simulink library "ddm"  (R2021b)
settings: Solver=VariableStepAuto  StartTime=0.0  StopTime=10.0  RelTol=1e-3
undefined symbols (not defined in the file or in its folder): ENUM_ADASACCSTA_ERROR, ENUM_ADASACCSTA_OFF, ENUM_ADASACCSTA_STANDBY, ENUM_ADASISASTA_OFF, ENUM_ALLOWMOV_ALLOWREADY, ENUM_APS, ENUM_BRKSTA_ERROR, ENUM_BRKSTA_OFF, ENUM_BRKSTA_ON, ENUM_BRKSW_INVALID, ENUM_BRKSW_OFF, ENUM_BRKSW_ON, ENUM_CHGPREACTERRSTA_OBCPRE, ENUM_DCDCFAULTSTA_ANYFAULTLV1, ENUM_DCDCFAULTSTA_ANYFAULTLV2, ENUM_DRIVETRAIN_AWD, ENUM_DRIVETRAIN_FWD, ENUM_DRIVETRAIN_RWD, ENUM_DRSEATSTA_INVALID, ENUM_EDUDRTSTA_NORMAL, ENUM_EPBSTA_APPLIED, ENUM_EPBSTA_RELEASED, ENUM_HVBATTREADYPRE_READY, ENUM_MCUWARN_LV0, ENUM_MCUWARN_LV1, ENUM_MCUWARN_LV2, ENUM_MCUWARN_LV3, ENUM_MCUWARN_NOERROR, ENUM_OBCFAULTSTA_ANYFAULT, ENUM_PAS_R2F2, ENUM_PDFAULT_BATTPDFAIL, ENUM_PDFAULT_DCDCDISABLE, ENUM_PDFAULT_MCUDISABLE, ENUM_PDFAULT_MCUDISCHRG, ENUM_POWERSTA_OFF, ENUM_POWERSTA_ON, ENUM_POWERSTA_READY, ENUM_POWERSTA_STANDBY, ENUM_PRESSINDI_LOW, ENUM_PUFAULT_BATTUPFAIL, ENUM_PUFAULT_DCDCENABLEFAIL, ENUM_PUFAULT_PRECHRGCHKFAIL, ENUM_PUFAULT_SAFETYCHKFAIL, ENUM_PUSTATE_COMPLETED, ENUM_PWRSTASW_OFF, ENUM_PWRSTASW_OFFA, ENUM_PWRSTASW_OFFCHVCHRG, ENUM_PWRSTASW_OFFCLVCHRG, ENUM_PWRSTASW_ON, ENUM_PWRSTASW_ONHVCHRG, ENUM_PWRSTASW_READY, ENUM_PWRSTASW_STANDBY, ENUM_RANGESTA_12IN, ENUM_SHIFTCOMMAND_D, ENUM_SHIFTCOMMAND_N, ENUM_SHIFTCOMMAND_P, ENUM_SHIFTCOMMAND_R, ENUM_VEHMALFUNLV_2ND, ENUM_VEHMALFUNLV_3RD, ENUM_VEHMALFUNLV_4TH ... (+835)
libraries: hcu_lib x750, $bdroot x12, simulink x5
(part 18 of 28)

== system ddm/DDM/DDM/PMM/Fault level/Fault level 1 subsystem error ==
  note: Diagnostics and Fault Handling
  note: Release Condition After Failure Decision
  note: Test Detection Criteria
  note: Test Pass Criteria
  note: Fail Safe Operation After Failure Decision
  note: Release Condition During Failure Detection
  note: Fail Safe Operation During Failure Detection
  task_time_s : Inport
  VPMM_PowerSta_enum : Inport  Port=2
  VPMM_PwrStaSW_enum : Inport  Port=3
  VDDM_C3BMS6LCCFS_flg : Inport  Port=4
  VDDM_C3CCU2LCCFS_flg : Inport  Port=5
  VDDM_MCUF1NoComCFS_flg : Inport  Port=6
  VDDM_MCUR1NoComCFS_flg : Inport  Port=7
  VINP_BMSWarn1_flg : Inport  Port=8
  VINP_BMSWarn2_flg : Inport  Port=9
  VINP_BMSWarn3_flg : Inport  Port=10
  VINP_DCDCFaultSta_enum : Inport  Port=11
  VINP_MCUWarnF_enum : Inport  Port=12
  VINP_MCUWarnR_enum : Inport  Port=13
  VINP_OBCFaultSta_enum : Inport  Port=14
  VPMM_DrivetrainSelect_enum : Inport  Port=15
  DTC_clear_request : Inport  Port=16
  No_CAN3_BUS_OFF : Inport  Port=17
  Constant : Constant  Value=KDDM_Lv1ErrDetTO_s
  Constant1 : Constant  Value=KDDM_Lv1ErrPassTO_s
  Constant{5,10,42,47} (4 alike) : Constant  Value=ENUM_MCUWARN_LV0
  Constant{6,11,43,49} (4 alike) : Constant  Value=ENUM_DRIVETRAIN_AWD
  Constant12 : Constant  Value=KDDM_Lv1ErrDTC_cnt
  Constant13 : Constant  Value=KDDM_Lv1ErrDetSW_flg
  Constant14 : Constant  Value=KDDM_Lv1ErrPassSW_flg
  Constant{15,21,25,27} (4 alike) : Constant  Value=FALSE
  Constant18 : Constant  Value=KDDM_Lv1ErrPassTO_s
  Constant2 : Constant  Value=KDDM_Lv1ErrCFSSW_flg
  Constant24 : Constant  Value=TRUE
  Constant26 : Constant  Value=ENUM_PWRSTASW_OFF
  Constant3 : Constant  Value=TRUE
  Constant36 : Constant  Value=ENUM_DCDCFAULTSTA_ANYFAULTLV1
  Constant37 : Constant  Value=ENUM_OBCFAULTSTA_ANYFAULT
  Constant38 : Constant  Value=ENUM_PWRSTASW_OFF
  Constant39 : Constant  Value=TRUE
  Constant4 : Constant  Value=ENUM_POWERSTA_OFF
  Constant40 : Constant  Value=KDDM_Lv1ErrDTC_cnt
  Constant44 : Constant  Value=ENUM_DRIVETRAIN_FWD
  Constant45 : Constant  Value=ENUM_DRIVETRAIN_RWD
  Constant50 : Constant  Value=ENUM_DCDCFAULTSTA_ANYFAULTLV1
  Constant51 : Constant  Value=ENUM_OBCFAULTSTA_ANYFAULT
  Constant7 : Constant  Value=ENUM_DRIVETRAIN_FWD
  Constant8 : Constant  Value=ENUM_DRIVETRAIN_RWD
  Constant9 : Constant  Value=KDDM_Lv1ErrDFSSW_flg
  DTC_Couter : hcu_lib/Basic_Blocks/DTC_Couter
  DTC_Info : hcu_lib/Basic_Blocks/DTC_Info
  Data Type Conversion1 : DataTypeConversion  OutDataTypeStr=uint8
  Equal : RelationalOperator  Operator=~=  OutDataTypeStr=boolean  RndMeth=Simplest
  Equal{1,4..9,14..21,25..26} (17 alike) : RelationalOperator  Operator===  OutDataTypeStr=boolean  RndMeth=Simplest
  Equal2 : RelationalOperator  Operator=~=  OutDataTypeStr=boolean  RndMeth=Simplest
  Equal3 : RelationalOperator  OutDataTypeStr=boolean  RndMeth=Simplest
  Goto24 : Goto  Commented=on  GotoTag=VDDM_EDriveSysErrVCUErr_flg
  Logical Operator{1,4..7,9..10,21,27..28} (10 alike) : Logic  Operator=NOT  AllPortsSameDT=off  OutDataTypeStr=boolean
  Logical Operator11 : Logic  Operator=OR  Inputs=7  AllPortsSameDT=off  OutDataTypeStr=boolean
  Logical Operator{12..13,15..16,18,22,24} (7 alike) : Logic  AllPortsSameDT=off  OutDataTypeStr=boolean
  Logical Operator{8,14,17,23,25,29..30} (7 alike) : Logic  Operator=OR  AllPortsSameDT=off  OutDataTypeStr=boolean
  Logical Operator19 : Logic  Inputs=3  AllPortsSameDT=off  OutDataTypeStr=boolean
  Logical Operator2 : Logic  Inputs=6  AllPortsSameDT=off  OutDataTypeStr=boolean
  Logical Operator20 : Logic  Operator=OR  Inputs=7  AllPortsSameDT=off  OutDataTypeStr=boolean
  Logical Operator26 : Logic  Inputs=6  AllPortsSameDT=off  OutDataTypeStr=boolean
  Logical Operator3 : Logic  Operator=OR  Inputs=3  AllPortsSameDT=off  OutDataTypeStr=boolean
  Relay : Relay  OnSwitchValue=ONE_INT  OffSwitchValue=ZERO_INT
  SR_Latch1 : Subsystem  mask(SR_Latch){}
      mask help: SR latch function.
  SR_Latch3 : hcu_lib/Basic_Blocks/SR_Latch
  SR_Latch4 : hcu_lib/Basic_Blocks/SR_Latch
  Switch{,2,4..6} (5 alike) : Switch  Criteria=u2 ~= 0
  Test Detection Criteria : hcu_lib/Basic_Blocks/Test Detection Criteria
  Timer1 : hcu_lib/Basic_Blocks/Timer
  VDDM_Lv1ErrDTC_raw32 : Outport
  wires:
  Logical Operator12/1 -> [VDDM_Lv1ErrDFS_flg]  "VDDM_Lv1ErrDFS_flg"
  Constant12/1 -> DTC_Couter/3
  Constant14/1 -> Logical Operator15/2
  Constant2/1 -> Logical Operator18/2
  DTC_Couter/1 -> SR_Latch4/1
  [VDDM_Lv1ErrDet_flg] -> Logical Operator19/1
  [DTC_clear_request] -> Logical Operator3/3
  Logical Operator18/1 -> [VDDM_Lv1ErrCFS_flg]  "VDDM_Lv1ErrCFS_flg"
  [DTC_clear_request] -> Logical Operator21/1
  [VDDM_Lv1ErrCFSRls_flg] -> Logical Operator29/1
  SR_Latch4/1 -> Logical Operator18/1
  [VDDM_Lv1ErrPass_flg] -> Logical Operator3/1
  DTC_Couter/2 -> Data Type Conversion1/1
  Logical Operator21/1 -> Logical Operator19/3
  Relay/1 -> SR_Latch3/1
  Data Type Conversion1/1 -> [VDDM_Lv1ErrDTC_cnt]  "VDDM_Lv1ErrDTC_cnt"
  Logical Operator15/1 -> DTC_Couter/2
  [VDDM_Lv1ErrCFSRls_flg] -> Logical Operator3/2
  Logical Operator30/1 -> SR_Latch3/2
  [VDDM_Lv1ErrCFS_flg] -> Logical Operator30/1
  Logical Operator29/1 -> SR_Latch4/2
  Logical Operator3/1 -> Logical Operator15/1
  [DTC_clear_request] -> Logical Operator29/2
  [DTC_clear_request] -> Logical Operator30/2
  [VDDM_Lv1ErrDTC_cnt] -> Relay/1
  Constant9/1 -> Logical Operator12/1
  Constant13/1 -> Logical Operator19/2
  Logical Operator19/1 -> DTC_Couter/1
  SR_Latch3/1 -> Logical Operator12/2
  [VDDM_xxx_flg] -> SR_Latch1/2(reset)
  Constant15/1 -> Switch6/1
  Switch5/1 -> Switch6/3, [VDDM_xxx_flg]
  Switch6/1 -> Test Detection Criteria/1
  [DTC_clear_request] -> Switch6/2
  [DTC_clear_request] -> DTC_Info/4
  Constant/1 -> Test Detection Criteria/4
  [VDDM_Lv1ErrDet_flg] -> DTC_Info/1
  [VDDM_Lv1ErrCFS_flg] -> DTC_Info/3
  [VDDM_Lv1ErrPass_flg] -> DTC_Info/2
  DTC_Info/1 -> VDDM_Lv1ErrDTC_raw32/1  "VDDM_Lv1ErrDTC_raw32"
  [task_time_s] -> Timer1/3
  No_CAN3_BUS_OFF/1 -> [No_CAN3_BUS_OFF]
  DTC_clear_request/1 -> [DTC_clear_request]
  Logical Operator16/1 -> Logical Operator11/5
  Logical Operator13/1 -> Logical Operator11/4
  Equal8/1 -> Logical Operator13/1
  Logical Operator17/1 -> Logical Operator16/2
  Equal7/1 -> Logical Operator17/2
  Equal6/1 -> Logical Operator16/1
  Constant10/1 -> Equal6/2
  Constant5/1 -> Equal8/2
  Equal9/1 -> Logical Operator14/2
  Equal1/1 -> Logical Operator14/1
  Logical Operator14/1 -> Logical Operator13/2
  Constant11/1 -> Equal7/2
  [VPMM_DrivetrainSelect_enum] -> Equal5/2, Equal7/1
  Constant6/1 -> Equal9/2
  Constant7/1 -> Equal1/1
  [VINP_MCUWarnF_enum] -> Equal8/1
  Constant8/1 -> Equal5/1
  [VINP_MCUWarnR_enum] -> Equal6/1
  [VPMM_DrivetrainSelect_enum] -> Equal1/2, Equal9/1
  Equal5/1 -> Logical Operator17/1
  [VPMM_PwrStaSW_enum] -> Equal/1
  [VPMM_PowerSta_enum] -> Equal4/1
  Logical Operator28/1 -> Logical Operator26/5
  Equal17/1 -> Logical Operator25/1
  [VPMM_DrivetrainSelect_enum] -> Equal26/1, Equal16/2
  [VINP_MCUWarnR_enum] -> Equal18/1
  Constant45/1 -> Equal17/1
  [VINP_MCUWarnF_enum] -> Equal25/1
  Constant44/1 -> Equal16/1
  Constant43/1 -> Equal26/2
  Logical Operator22/1 -> Logical Operator20/4
  Constant39/1 -> Switch2/3
  Constant51/1 -> Equal21/2
  Logical Operator24/1 -> Logical Operator20/5
  [VPMM_DrivetrainSelect_enum] -> Equal19/1, Equal17/2
  Logical Operator5/1 -> Logical Operator26/6
  Constant50/1 -> Equal20/2
  [VDDM_C3CCU2LCCFS_flg] -> Logical Operator27/1
  [VDDM_MCUF1NoComCFS_flg] -> Logical Operator28/1
  Constant49/1 -> Equal19/2
  [VPMM_PwrStaSW_enum] -> Equal2/1
  Equal2/1 -> Logical Operator26/2
  [VDDM_MCUR1NoComCFS_flg] -> Logical Operator5/1
  Equal20/1 -> Logical Operator20/6
  Equal21/1 -> Logical Operator20/7
  Logical Operator23/1 -> Logical Operator22/2
  Logical Operator26/1 -> Switch2/2
  Equal16/1 -> Logical Operator23/1
  [VINP_OBCFaultSta_enum] -> Equal21/1
  Logical Operator20/1 -> Switch2/1
  Equal26/1 -> Logical Operator23/2
  [VINP_DCDCFaultSta_enum] -> Equal20/1
  Constant42/1 -> Equal25/2
  Logical Operator27/1 -> Logical Operator26/4
  [VINP_BMSWarn2_flg] -> Logical Operator20/2
  [VINP_BMSWarn1_flg] -> Logical Operator20/1
  [VINP_BMSWarn3_flg] -> Logical Operator20/3
  [VDDM_C3BMS6LCCFS_flg] -> Logical Operator4/1
  Logical Operator4/1 -> Logical Operator26/3
  Constant47/1 -> Equal18/2
  [No_CAN3_BUS_OFF] -> Logical Operator26/1
  Constant38/1 -> Equal2/2
  Equal18/1 -> Logical Operator24/1
  Equal19/1 -> Logical Operator25/2
  Logical Operator25/1 -> Logical Operator24/2
  Equal25/1 -> Logical Operator22/1
  Equal15/1 -> Logical Operator11/7
  Equal14/1 -> Logical Operator11/6
  [VINP_BMSWarn1_flg] -> Logical Operator11/1
  Logical Operator11/1 -> Switch5/1
  Constant37/1 -> Equal15/2
  [VINP_OBCFaultSta_enum] -> Equal15/1
  Constant36/1 -> Equal14/2
  [VINP_DCDCFaultSta_enum] -> Equal14/1
  [VINP_BMSWarn3_flg] -> Logical Operator11/3
  [VINP_BMSWarn2_flg] -> Logical Operator11/2
  Logical Operator10/1 -> Logical Operator2/6
  [VDDM_MCUR1NoComCFS_flg] -> Logical Operator10/1
  Logical Operator9/1 -> Logical Operator2/5
  [VDDM_MCUF1NoComCFS_flg] -> Logical Operator9/1
  [VDDM_C3CCU2LCCFS_flg] -> Logical Operator7/1
  Logical Operator7/1 -> Logical Operator2/4
  Constant4/1 -> Equal4/2
  [VDDM_Lv1ErrCFS_flg] -> Switch/2
  Switch2/1 -> Timer1/2, Logical Operator6/1
  Constant18/1 -> Equal3/2
  Logical Operator6/1 -> Timer1/1
  Constant24/1 -> Switch4/1
  Constant40/1 -> Test Detection Criteria/3
  Equal/1 -> Logical Operator2/2
  [task_time_s] -> Test Detection Criteria/2
  Logical Operator2/1 -> Switch5/2
  [VDDM_C3BMS6LCCFS_flg] -> Logical Operator1/1
  Switch4/1 -> [VDDM_Lv1ErrCFSRls_flg]  "VDDM_Lv1ErrCFSRls_flg"
  Constant27/1 -> Switch5/3
  Test Detection Criteria/1 -> [VDDM_Lv1ErrDet_flg]  "VDDM_Lv1ErrDet_flg"
  Constant26/1 -> Equal/2
  Logical Operator8/1 -> Switch4/2
  [No_CAN3_BUS_OFF] -> Logical Operator2/1
  Equal3/1 -> SR_Latch1/1(set)
  Logical Operator1/1 -> Logical Operator2/3
  Constant25/1 -> Switch4/3
  Timer1/1 -> Equal3/1
  SR_Latch1/1(latched) -> [VDDM_Lv1ErrPass_flg]  "VDDM_Lv1ErrPass_flg"
  Constant3/1 -> Switch/1
  [DTC_clear_request] -> Logical Operator8/2
  Switch/1 -> Goto24/1
  Constant21/1 -> Switch/3
  Constant1/1 -> Timer1/4
  Equal4/1 -> Logical Operator8/1
  VDDM_C3BMS6LCCFS_flg/1 -> [VDDM_C3BMS6LCCFS_flg]
  VINP_OBCFaultSta_enum/1 -> [VINP_OBCFaultSta_enum]
  VINP_MCUWarnF_enum/1 -> [VINP_MCUWarnF_enum]
  VINP_DCDCFaultSta_enum/1 -> [VINP_DCDCFaultSta_enum]
  VINP_BMSWarn3_flg/1 -> [VINP_BMSWarn3_flg]
  VINP_BMSWarn2_flg/1 -> [VINP_BMSWarn2_flg]
  VINP_BMSWarn1_flg/1 -> [VINP_BMSWarn1_flg]
  VDDM_MCUF1NoComCFS_flg/1 -> [VDDM_MCUF1NoComCFS_flg]
  VDDM_MCUR1NoComCFS_flg/1 -> [VDDM_MCUR1NoComCFS_flg]
  VINP_MCUWarnR_enum/1 -> [VINP_MCUWarnR_enum]
  VPMM_DrivetrainSelect_enum/1 -> [VPMM_DrivetrainSelect_enum]
  VDDM_C3CCU2LCCFS_flg/1 -> [VDDM_C3CCU2LCCFS_flg]
  VPMM_PowerSta_enum/1 -> [VPMM_PowerSta_enum]
  VPMM_PwrStaSW_enum/1 -> [VPMM_PwrStaSW_enum]
  task_time_s/1 -> [task_time_s]

== system ddm/DDM/DDM/PMM/Fault level/Fault level 2 subsystem error ==
  note: Diagnostics and Fault Handling
  note: Release Condition After Failure Decision
  note: Fail Safe Operation After Failure Decision
  note: Test Detection Criteria
  note: Fail Safe Operation During Failure Detection
  note: Release Condition During Failure Detection
  note: Test Pass Criteria
  task_time_s : Inport
  VPMM_PowerSta_enum : Inport  Port=2
  VPMM_PwrStaSW_enum : Inport  Port=3
  VDDM_C3BMS6LCCFS_flg : Inport  Port=4
  VDDM_C3CCU2LCCFS_flg : Inport  Port=5
  VDDM_MCUF1NoComCFS_flg : Inport  Port=6
  VDDM_MCUR1NoComCFS_flg : Inport  Port=7
  VINP_BMSWarn4_flg : Inport  Port=8
  VINP_BMSWarn5_flg : Inport  Port=9
  VINP_DCDCFaultSta_enum : Inport  Port=10
  VINP_MCUWarnF_enum : Inport  Port=11
  VINP_MCUWarnR_enum : Inport  Port=12
  VPMM_DrivetrainSelect_enum : Inport  Port=13
  DTC_clear_request : Inport  Port=14
  No_CAN3_BUS_OFF : Inport  Port=15
  Constant1 : Constant  Value=ENUM_PWRSTASW_OFF
  Constant{6,10,30,34} (4 alike) : Constant  Value=ENUM_MCUWARN_LV2
  Constant{7,11,31,35} (4 alike) : Constant  Value=ENUM_DRIVETRAIN_AWD
  Constant12 : Constant  Value=ENUM_DCDCFAULTSTA_ANYFAULTLV2
  Constant{2,13,29,37} (4 alike) : Constant  Value=ENUM_MCUWARN_LV1
  Constant{14,21,25,27} (4 alike) : Constant  Value=FALSE
  Constant15 : Constant  Value=KDDM_Lv2ErrDetSW_flg
  Constant16 : Constant  Value=KDDM_Lv2ErrPassSW_flg
  Constant19 : Constant  Value=KDDM_Lv2ErrPassTO_s
  Constant20 : Constant  Value=KDDM_Lv2ErrCFSSW_flg
  Constant22 : Constant  Value=TRUE
  Constant23 : Constant  Value=ENUM_POWERSTA_OFF
  Constant24 : Constant  Value=TRUE
  Constant26 : Constant  Value=ENUM_PWRSTASW_OFF
  Constant3 : Constant  Value=KDDM_Lv2ErrDetTO_s
  Constant32 : Constant  Value=ENUM_DRIVETRAIN_FWD
  Constant33 : Constant  Value=ENUM_DRIVETRAIN_RWD
  Constant36 : Constant  Value=ENUM_DCDCFAULTSTA_ANYFAULTLV2
  Constant39 : Constant  Value=TRUE
  Constant4 : Constant  Value=KDDM_Lv2ErrPassTO_s
  Constant40 : Constant  Value=KDDM_Lv2ErrDTC_cnt
  Constant46 : Constant  Value=KDDM_Lv2ErrDFSSW_flg
  Constant5 : Constant  Value=KDDM_Lv2ErrDTC_cnt
  Constant8 : Constant  Value=ENUM_DRIVETRAIN_FWD
  Constant9 : Constant  Value=ENUM_DRIVETRAIN_RWD
  DTC_Couter : hcu_lib/Basic_Blocks/DTC_Couter
  DTC_Info : hcu_lib/Basic_Blocks/DTC_Info
  Data Type Conversion1 : DataTypeConversion  OutDataTypeStr=uint8
  Equal : RelationalOperator  Operator=~=  OutDataTypeStr=boolean  RndMeth=Simplest
  Equal1 : RelationalOperator  Operator=~=  OutDataTypeStr=boolean  RndMeth=Simplest
  Equal{2,4..21} (19 alike) : RelationalOperator  Operator===  OutDataTypeStr=boolean  RndMeth=Simplest
  Equal3 : RelationalOperator  OutDataTypeStr=boolean  RndMeth=Simplest
  Goto24 : Goto  Commented=on  GotoTag=VDDM_EDriveSysErrVCUErr_flg
  Logical Operator{1,4..7,9..10,21,31..32} (10 alike) : Logic  Operator=NOT  AllPortsSameDT=off  OutDataTypeStr=boolean
  Logical Operator11 : Logic  Operator=OR  Inputs=5  AllPortsSameDT=off  OutDataTypeStr=boolean
  Logical Operator{12..13,15..16,18,22,24} (7 alike) : Logic  AllPortsSameDT=off  OutDataTypeStr=boolean
  Logical Operator{8,14,17,23,25,27..30,33..34} (11 alike) : Logic  Operator=OR  AllPortsSameDT=off  OutDataTypeStr=boolean
  Logical Operator19 : Logic  Inputs=3  AllPortsSameDT=off  OutDataTypeStr=boolean
  Logical Operator2 : Logic  Inputs=6  AllPortsSameDT=off  OutDataTypeStr=boolean
  Logical Operator20 : Logic  Operator=OR  Inputs=5  AllPortsSameDT=off  OutDataTypeStr=boolean
  Logical Operator26 : Logic  Inputs=6  AllPortsSameDT=off  OutDataTypeStr=boolean
  Logical Operator3 : Logic  Operator=OR  Inputs=3  AllPortsSameDT=off  OutDataTypeStr=boolean
  Relay : Relay  OnSwitchValue=ONE_INT  OffSwitchValue=ZERO_INT
  SR_Latch1 : Subsystem  mask(SR_Latch){}
      mask help: SR latch function.
  SR_Latch3 : hcu_lib/Basic_Blocks/SR_Latch
  SR_Latch4 : hcu_lib/Basic_Blocks/SR_Latch
  Switch{,2,4..6} (5 alike) : Switch  Criteria=u2 ~= 0
  Test Detection Criteria : hcu_lib/Basic_Blocks/Test Detection Criteria
  Timer1 : hcu_lib/Basic_Blocks/Timer
  VDDM_Lv2ErrDTC_raw32 : Outport
  wires:
  [VDDM_Lv2ErrDTC_cnt] -> Relay/1
  SR_Latch4/1 -> Logical Operator18/1
  [VDDM_Lv2ErrDet_flg] -> Logical Operator19/1
  [VDDM_Lv2ErrPass_flg] -> Logical Operator3/1
  Logical Operator34/1 -> SR_Latch3/2
  Logical Operator21/1 -> Logical Operator19/3
  [DTC_clear_request] -> Logical Operator21/1
  Logical Operator15/1 -> DTC_Couter/2
  [DTC_clear_request] -> Logical Operator3/3
  [DTC_clear_request] -> Logical Operator34/2
  [VDDM_Lv2ErrCFS_flg] -> Logical Operator34/1
  [DTC_clear_request] -> Logical Operator33/2
  Constant15/1 -> Logical Operator19/2
  Logical Operator33/1 -> SR_Latch4/2
  Relay/1 -> SR_Latch3/1
  SR_Latch3/1 -> Logical Operator12/2
  Logical Operator19/1 -> DTC_Couter/1
  Logical Operator12/1 -> [VDDM_Lv2ErrDFS_flg]  "VDDM_Lv2ErrDFS_flg"
  Constant5/1 -> DTC_Couter/3
  [VDDM_Lv2ErrCFSRls_flg] -> Logical Operator3/2
  Constant20/1 -> Logical Operator18/2
  [VDDM_Lv2ErrCFSRls_flg] -> Logical Operator33/1
  Logical Operator18/1 -> [VDDM_Lv2ErrCFS_flg]  "VDDM_Lv2ErrCFS_flg"
  DTC_Couter/1 -> SR_Latch4/1
  Logical Operator3/1 -> Logical Operator15/1
  DTC_Couter/2 -> Data Type Conversion1/1
  Constant46/1 -> Logical Operator12/1
  Data Type Conversion1/1 -> [VDDM_Lv2ErrDTC_cnt]  "VDDM_Lv2ErrDTC_cnt"
  Constant16/1 -> Logical Operator15/2
  [VDDM_xxx_flg] -> SR_Latch1/2(reset)
  Constant14/1 -> Switch6/1
  Switch5/1 -> Switch6/3, [VDDM_xxx_flg]
  Switch6/1 -> Test Detection Criteria/1
  [DTC_clear_request] -> Switch6/2
  [DTC_clear_request] -> DTC_Info/4
  Constant3/1 -> Test Detection Criteria/4
  [VDDM_Lv2ErrDet_flg] -> DTC_Info/1
  [VDDM_Lv2ErrCFS_flg] -> DTC_Info/3
  [VDDM_Lv2ErrPass_flg] -> DTC_Info/2
  DTC_Info/1 -> VDDM_Lv2ErrDTC_raw32/1  "VDDM_Lv2ErrDTC_raw32"
  [task_time_s] -> Timer1/3
  No_CAN3_BUS_OFF/1 -> [No_CAN3_BUS_OFF]
  DTC_clear_request/1 -> [DTC_clear_request]
  Equal21/1 -> Logical Operator23/2
  Equal2/1 -> Logical Operator23/1
  [VDDM_MCUF1NoComCFS_flg] -> Logical Operator32/1
  Logical Operator31/1 -> Logical Operator26/4
  [VINP_BMSWarn4_flg] -> Logical Operator20/1
  Logical Operator24/1 -> Logical Operator20/4
  [VINP_BMSWarn5_flg] -> Logical Operator20/2
  Logical Operator22/1 -> Logical Operator20/3
  Constant12/1 -> Equal17/2
  [No_CAN3_BUS_OFF] -> Logical Operator26/1
  [VPMM_DrivetrainSelect_enum] -> Equal16/1, Equal5/2
  Constant9/1 -> Equal5/1
  Constant7/1 -> Equal21/2
  Constant11/1 -> Equal16/2
  [VINP_MCUWarnR_enum] -> Equal6/1, Equal18/2
  Logical Operator25/1 -> Logical Operator24/2
  Logical Operator23/1 -> Logical Operator22/2
  Constant8/1 -> Equal2/1
  [VPMM_DrivetrainSelect_enum] -> Equal21/1, Equal2/2
  Constant1/1 -> Equal1/2
  Equal16/1 -> Logical Operator25/2
  Constant6/1 -> Equal20/2
  [VDDM_C3CCU2LCCFS_flg] -> Logical Operator31/1
  Logical Operator5/1 -> Logical Operator26/6
  [VDDM_MCUR1NoComCFS_flg] -> Logical Operator5/1
  Logical Operator4/1 -> Logical Operator26/3
  Logical Operator32/1 -> Logical Operator26/5
  Logical Operator26/1 -> Switch2/2
  Equal5/1 -> Logical Operator25/1
  [VDDM_C3BMS6LCCFS_flg] -> Logical Operator4/1
  Equal17/1 -> Logical Operator20/5
  Equal1/1 -> Logical Operator26/2
  Constant10/1 -> Equal6/2
  [VINP_DCDCFaultSta_enum] -> Equal17/1
  Logical Operator20/1 -> Switch2/1
  [VINP_MCUWarnF_enum] -> Equal20/1, Equal19/2
  Constant2/1 -> Equal19/1
  Equal19/1 -> Logical Operator27/1
  Equal20/1 -> Logical Operator27/2
  Logical Operator27/1 -> Logical Operator22/1
  Constant13/1 -> Equal18/1
  Equal18/1 -> Logical Operator28/1
  Equal6/1 -> Logical Operator28/2
  Logical Operator28/1 -> Logical Operator24/1
  [VPMM_PwrStaSW_enum] -> Equal1/1
  [VPMM_PwrStaSW_enum] -> Equal/1
  [VPMM_PowerSta_enum] -> Equal4/1
  Logical Operator30/1 -> Logical Operator16/1
  Equal12/1 -> Logical Operator30/2
  Equal15/1 -> Logical Operator30/1
  Constant37/1 -> Equal15/1
  Logical Operator29/1 -> Logical Operator13/1
  Equal8/1 -> Logical Operator29/2
  Equal7/1 -> Logical Operator29/1
  Constant29/1 -> Equal7/1
  Constant4/1 -> Timer1/4
  [VINP_MCUWarnF_enum] -> Equal7/2, Equal8/1
  Logical Operator11/1 -> Switch5/1
  Switch4/1 -> [VDDM_Lv2ErrCFSRls_flg]  "VDDM_Lv2ErrCFSRls_flg"
  [VINP_DCDCFaultSta_enum] -> Equal14/1
  Constant34/1 -> Equal12/2
  Constant23/1 -> Equal4/2
  Equal/1 -> Logical Operator2/2
  Constant25/1 -> Switch4/3
  [VDDM_Lv2ErrCFS_flg] -> Switch/2
  Equal3/1 -> SR_Latch1/1(set)
  Equal14/1 -> Logical Operator11/5
  [VDDM_C3BMS6LCCFS_flg] -> Logical Operator1/1
  Equal11/1 -> Logical Operator17/1
  Switch/1 -> Goto24/1
  Constant40/1 -> Test Detection Criteria/3
  Equal4/1 -> Logical Operator8/1
  [DTC_clear_request] -> Logical Operator8/2
  Timer1/1 -> Equal3/1
  Constant19/1 -> Equal3/2
  Logical Operator2/1 -> Switch5/2
  Constant24/1 -> Switch4/1
  Logical Operator9/1 -> Logical Operator2/5
  Logical Operator1/1 -> Logical Operator2/3
  Switch2/1 -> Logical Operator6/1, Timer1/2
  [VDDM_MCUR1NoComCFS_flg] -> Logical Operator10/1
  Logical Operator8/1 -> Switch4/2
  Logical Operator10/1 -> Logical Operator2/6
  [VDDM_C3CCU2LCCFS_flg] -> Logical Operator7/1
  Constant30/1 -> Equal8/2
  Constant27/1 -> Switch5/3
  Equal13/1 -> Logical Operator17/2
  Constant26/1 -> Equal/2
  [VPMM_DrivetrainSelect_enum] -> Equal10/2, Equal9/1
  Constant32/1 -> Equal10/1
  Logical Operator14/1 -> Logical Operator13/2
  Logical Operator17/1 -> Logical Operator16/2
  Constant22/1 -> Switch/1
  [VINP_MCUWarnR_enum] -> Equal15/2, Equal12/1
  Constant35/1 -> Equal13/2
  Constant31/1 -> Equal9/2
  Constant33/1 -> Equal11/1
  [VPMM_DrivetrainSelect_enum] -> Equal11/2, Equal13/1
  [No_CAN3_BUS_OFF] -> Logical Operator2/1
  Constant36/1 -> Equal14/2
  Logical Operator6/1 -> Timer1/1
  Logical Operator13/1 -> Logical Operator11/3
  [VINP_BMSWarn5_flg] -> Logical Operator11/2
  Logical Operator16/1 -> Logical Operator11/4
  [VINP_BMSWarn4_flg] -> Logical Operator11/1
  [task_time_s] -> Test Detection Criteria/2
  Logical Operator7/1 -> Logical Operator2/4
  Constant21/1 -> Switch/3
  Test Detection Criteria/1 -> [VDDM_Lv2ErrDet_flg]  "VDDM_Lv2ErrDet_flg"
  Constant39/1 -> Switch2/3
  SR_Latch1/1(latched) -> [VDDM_Lv2ErrPass_flg]  "VDDM_Lv2ErrPass_flg"
  [VDDM_MCUF1NoComCFS_flg] -> Logical Operator9/1
  Equal10/1 -> Logical Operator14/1
  Equal9/1 -> Logical Operator14/2
  VDDM_C3BMS6LCCFS_flg/1 -> [VDDM_C3BMS6LCCFS_flg]
  VINP_BMSWarn4_flg/1 -> [VINP_BMSWarn4_flg]
  VINP_BMSWarn5_flg/1 -> [VINP_BMSWarn5_flg]
  task_time_s/1 -> [task_time_s]
  VPMM_PwrStaSW_enum/1 -> [VPMM_PwrStaSW_enum]
  VPMM_PowerSta_enum/1 -> [VPMM_PowerSta_enum]
  VDDM_C3CCU2LCCFS_flg/1 -> [VDDM_C3CCU2LCCFS_flg]
  VPMM_DrivetrainSelect_enum/1 -> [VPMM_DrivetrainSelect_enum]
  VINP_MCUWarnR_enum/1 -> [VINP_MCUWarnR_enum]
  VDDM_MCUR1NoComCFS_flg/1 -> [VDDM_MCUR1NoComCFS_flg]
  VDDM_MCUF1NoComCFS_flg/1 -> [VDDM_MCUF1NoComCFS_flg]
  VINP_DCDCFaultSta_enum/1 -> [VINP_DCDCFaultSta_enum]
  VINP_MCUWarnF_enum/1 -> [VINP_MCUWarnF_enum]

== system ddm/DDM/DDM/PMM/Fault level/Fault level 3 subsystem error ==
  note: Diagnostics and Fault Handling
  note: Release Condition After Failure Decision
  note: Fail Safe Operation After Failure Decision
  note: Test Detection Criteria
  note: Fail Safe Operation During Failure Detection
  note: Release Condition During Failure Detection
  note: Test Pass Criteria
  task_time_s : Inport
  VPMM_PowerSta_enum : Inport  Port=2
  VPMM_PwrStaSW_enum : Inport  Port=3
  VDDM_C3BMS6LCCFS_flg : Inport  Port=4
  VDDM_MCUF1NoComCFS_flg : Inport  Port=5
  VDDM_MCUR1NoComCFS_flg : Inport  Port=6
  VINP_BMSWarn6_flg : Inport  Port=7
  VINP_MCUWarnF_enum : Inport  Port=8
  VINP_MCUWarnR_enum : Inport  Port=9
  VPMM_DrivetrainSelect_enum : Inport  Port=10
  DTC_clear_request : Inport  Port=11
  No_CAN3_BUS_OFF : Inport  Port=12
  Constant{1,8,30,34} (4 alike) : Constant  Value=ENUM_MCUWARN_LV3
  Constant10 : Constant  Value=KDDM_Lv3ErrDetSW_flg
  Constant11 : Constant  Value=KDDM_Lv3ErrPassSW_flg
  Constant{12,21,25,27} (4 alike) : Constant  Value=FALSE
  Constant15 : Constant  Value=KDDM_Lv3ErrCFSSW_flg
  Constant16 : Constant  Value=TRUE
  Constant18 : Constant  Value=KDDM_Lv3ErrPassTO_s
  Constant19 : Constant  Value=ENUM_POWERSTA_OFF
  Constant{2,9,31,35} (4 alike) : Constant  Value=ENUM_DRIVETRAIN_AWD
  Constant20 : Constant  Value=KDDM_Lv3ErrDFSSW_flg
  Constant24 : Constant  Value=TRUE
  Constant26 : Constant  Value=ENUM_PWRSTASW_OFF
  Constant3 : Constant  Value=KDDM_Lv3ErrDetTO_s
  Constant32 : Constant  Value=ENUM_DRIVETRAIN_FWD
  Constant33 : Constant  Value=ENUM_DRIVETRAIN_RWD
  Constant38 : Constant  Value=ENUM_PWRSTASW_OFF
  Constant39 : Constant  Value=TRUE
  Constant4 : Constant  Value=KDDM_Lv3ErrPassTO_s
  Constant40 : Constant  Value=KDDM_Lv3ErrDTC_cnt
  Constant5 : Constant  Value=KDDM_Lv3ErrDTC_cnt
  Constant6 : Constant  Value=ENUM_DRIVETRAIN_FWD
  Constant7 : Constant  Value=ENUM_DRIVETRAIN_RWD
  DTC_Couter : hcu_lib/Basic_Blocks/DTC_Couter
  DTC_Info : hcu_lib/Basic_Blocks/DTC_Info
  Data Type Conversion1 : DataTypeConversion  OutDataTypeStr=uint8
  Equal : RelationalOperator  Operator=~=  OutDataTypeStr=boolean  RndMeth=Simplest
  Equal{1,4..15} (13 alike) : RelationalOperator  Operator===  OutDataTypeStr=boolean  RndMeth=Simplest
  Equal2 : RelationalOperator  Operator=~=  OutDataTypeStr=boolean  RndMeth=Simplest
  Equal3 : RelationalOperator  OutDataTypeStr=boolean  RndMeth=Simplest
  Goto24 : Goto  Commented=on  GotoTag=VDDM_EDriveSysErrVCUErr_flg
  Logical Operator{1,4..6,9..10,21,26} (8 alike) : Logic  Operator=NOT  AllPortsSameDT=off  OutDataTypeStr=boolean
  Logical Operator11 : Logic  Operator=OR  Inputs=3  AllPortsSameDT=off  OutDataTypeStr=boolean
  Logical Operator{12..13,15..16,18,20,23} (7 alike) : Logic  AllPortsSameDT=off  OutDataTypeStr=boolean
  Logical Operator{8,14,17,22,24,27..28} (7 alike) : Logic  Operator=OR  AllPortsSameDT=off  OutDataTypeStr=boolean
  Logical Operator19 : Logic  Inputs=3  AllPortsSameDT=off  OutDataTypeStr=boolean
  Logical Operator2 : Logic  Inputs=5  AllPortsSameDT=off  OutDataTypeStr=boolean
  Logical Operator25 : Logic  Inputs=5  AllPortsSameDT=off  OutDataTypeStr=boolean
  Logical Operator3 : Logic  Operator=OR  Inputs=3  AllPortsSameDT=off  OutDataTypeStr=boolean
  Logical Operator7 : Logic  Operator=OR  Inputs=3  AllPortsSameDT=off  OutDataTypeStr=boolean
  Relay : Relay  OnSwitchValue=ONE_INT  OffSwitchValue=ZERO_INT
  SR_Latch1 : Subsystem  mask(SR_Latch){}
      mask help: SR latch function.
  SR_Latch3 : hcu_lib/Basic_Blocks/SR_Latch
  SR_Latch4 : hcu_lib/Basic_Blocks/SR_Latch
  Switch{,2,4..6} (5 alike) : Switch  Criteria=u2 ~= 0
  Test Detection Criteria : hcu_lib/Basic_Blocks/Test Detection Criteria
  Timer1 : hcu_lib/Basic_Blocks/Timer
  VDDM_Lv3ErrDTC_raw32 : Outport
  wires:
  SR_Latch4/1 -> Logical Operator18/1
  Constant5/1 -> DTC_Couter/3
  Logical Operator3/1 -> Logical Operator15/1
  DTC_Couter/1 -> SR_Latch4/1
  Logical Operator15/1 -> DTC_Couter/2
  Constant10/1 -> Logical Operator19/2
  Logical Operator28/1 -> SR_Latch3/2
  [DTC_clear_request] -> Logical Operator27/2
  Data Type Conversion1/1 -> [VDDM_Lv3ErrDTC_cnt]  "VDDM_Lv3ErrDTC_cnt"
  SR_Latch3/1 -> Logical Operator12/2
  Constant15/1 -> Logical Operator18/2
  DTC_Couter/2 -> Data Type Conversion1/1
  Logical Operator12/1 -> [VDDM_Lv3ErrDFS_flg]  "VDDM_Lv3ErrDFS_flg"
  [VDDM_Lv3ErrCFSRls_flg] -> Logical Operator27/1
  Constant11/1 -> Logical Operator15/2
  [VDDM_Lv3ErrCFSRls_flg] -> Logical Operator3/2
  Logical Operator27/1 -> SR_Latch4/2
  Logical Operator18/1 -> [VDDM_Lv3ErrCFS_flg]  "VDDM_Lv3ErrCFS_flg"
  Logical Operator19/1 -> DTC_Couter/1
  [DTC_clear_request] -> Logical Operator28/2
  Constant20/1 -> Logical Operator12/1
  Relay/1 -> SR_Latch3/1
  [VDDM_Lv3ErrCFS_flg] -> Logical Operator28/1
  [VDDM_Lv3ErrDTC_cnt] -> Relay/1
  [VDDM_Lv3ErrDet_flg] -> Logical Operator19/1
  [DTC_clear_request] -> Logical Operator21/1
  [VDDM_Lv3ErrPass_flg] -> Logical Operator3/1
  [DTC_clear_request] -> Logical Operator3/3
  Logical Operator21/1 -> Logical Operator19/3
  [VDDM_xxx_flg] -> SR_Latch1/2(reset)
  Constant12/1 -> Switch6/1
  Switch5/1 -> Switch6/3, [VDDM_xxx_flg]
  Switch6/1 -> Test Detection Criteria/1
  [DTC_clear_request] -> Switch6/2
  [DTC_clear_request] -> DTC_Info/4
  Constant3/1 -> Test Detection Criteria/4
  [VDDM_Lv3ErrDet_flg] -> DTC_Info/1
  [VDDM_Lv3ErrCFS_flg] -> DTC_Info/3
  [VDDM_Lv3ErrPass_flg] -> DTC_Info/2
  DTC_Info/1 -> VDDM_Lv3ErrDTC_raw32/1  "VDDM_Lv3ErrDTC_raw32"
  [task_time_s] -> Timer1/3
  No_CAN3_BUS_OFF/1 -> [No_CAN3_BUS_OFF]
  DTC_clear_request/1 -> [DTC_clear_request]
  Logical Operator20/1 -> Logical Operator7/2
  Logical Operator23/1 -> Logical Operator7/3
  Equal15/1 -> Logical Operator22/2
  Equal1/1 -> Logical Operator22/1
  [VPMM_DrivetrainSelect_enum] -> Equal5/2, Equal7/1
  Constant7/1 -> Equal5/1
  Constant2/1 -> Equal15/2
  Constant9/1 -> Equal7/2
  [VINP_MCUWarnR_enum] -> Equal6/1
  Logical Operator24/1 -> Logical Operator23/2
  Logical Operator22/1 -> Logical Operator20/2
  Constant6/1 -> Equal1/1
  Equal6/1 -> Logical Operator23/1
  [VPMM_DrivetrainSelect_enum] -> Equal1/2, Equal15/1
  Equal14/1 -> Logical Operator20/1
  Constant1/1 -> Equal14/2
  Equal7/1 -> Logical Operator24/2
  Equal5/1 -> Logical Operator24/1
  Constant8/1 -> Equal6/2
  [VINP_MCUWarnF_enum] -> Equal14/1
  [VPMM_PwrStaSW_enum] -> Equal2/1
  [VPMM_PwrStaSW_enum] -> Equal/1
  [VPMM_PowerSta_enum] -> Equal4/1
  Logical Operator25/1 -> Switch2/2
  Logical Operator26/1 -> Logical Operator25/4
  Equal2/1 -> Logical Operator25/2
  Logical Operator5/1 -> Logical Operator25/5
  Logical Operator4/1 -> Logical Operator25/3
  [VDDM_MCUR1NoComCFS_flg] -> Logical Operator5/1
  Constant38/1 -> Equal2/2
  [VDDM_C3BMS6LCCFS_flg] -> Logical Operator4/1
  [No_CAN3_BUS_OFF] -> Logical Operator25/1
  [VDDM_MCUF1NoComCFS_flg] -> Logical Operator26/1
  Logical Operator7/1 -> Switch2/1
  [VINP_BMSWarn6_flg] -> Logical Operator7/1
  Constant4/1 -> Timer1/4
  [VINP_MCUWarnF_enum] -> Equal8/1
  Logical Operator11/1 -> Switch5/1
  Switch4/1 -> [VDDM_Lv3ErrCFSRls_flg]  "VDDM_Lv3ErrCFSRls_flg"
  Constant19/1 -> Equal4/2
  Constant34/1 -> Equal12/2
  Equal/1 -> Logical Operator2/2
  Constant25/1 -> Switch4/3
  [VDDM_Lv3ErrCFS_flg] -> Switch/2
  Equal3/1 -> SR_Latch1/1(set)
  [VDDM_C3BMS6LCCFS_flg] -> Logical Operator1/1
  Equal11/1 -> Logical Operator17/1
  Switch/1 -> Goto24/1
  Constant40/1 -> Test Detection Criteria/3
  Equal4/1 -> Logical Operator8/1
  [DTC_clear_request] -> Logical Operator8/2
  Timer1/1 -> Equal3/1
  Constant26/1 -> Equal/2
  Constant18/1 -> Equal3/2
  Logical Operator2/1 -> Switch5/2
  Equal13/1 -> Logical Operator17/2
  Constant24/1 -> Switch4/1
  Logical Operator9/1 -> Logical Operator2/4
  Logical Operator1/1 -> Logical Operator2/3
  Switch2/1 -> Timer1/2, Logical Operator6/1
  Constant27/1 -> Switch5/3
  [VDDM_MCUR1NoComCFS_flg] -> Logical Operator10/1
  Logical Operator8/1 -> Switch4/2
  Logical Operator10/1 -> Logical Operator2/5
  Constant30/1 -> Equal8/2
  Equal8/1 -> Logical Operator13/1
  [VPMM_DrivetrainSelect_enum] -> Equal9/1, Equal10/2
  Equal12/1 -> Logical Operator16/1
  Constant32/1 -> Equal10/1
  Logical Operator14/1 -> Logical Operator13/2
  Logical Operator17/1 -> Logical Operator16/2
  Constant16/1 -> Switch/1
  [VINP_MCUWarnR_enum] -> Equal12/1
  Constant35/1 -> Equal13/2
  Constant31/1 -> Equal9/2
  Constant33/1 -> Equal11/1
  [VPMM_DrivetrainSelect_enum] -> Equal13/1, Equal11/2
  [No_CAN3_BUS_OFF] -> Logical Operator2/1
  Logical Operator6/1 -> Timer1/1
  Logical Operator13/1 -> Logical Operator11/2
  Logical Operator16/1 -> Logical Operator11/3
  [task_time_s] -> Test Detection Criteria/2
  Constant21/1 -> Switch/3
  Test Detection Criteria/1 -> [VDDM_Lv3ErrDet_flg]  "VDDM_Lv3ErrDet_flg"
  Constant39/1 -> Switch2/3
  SR_Latch1/1(latched) -> [VDDM_Lv3ErrPass_flg]  "VDDM_Lv3ErrPass_flg"
  [VDDM_MCUF1NoComCFS_flg] -> Logical Operator9/1
  Equal10/1 -> Logical Operator14/1
  Equal9/1 -> Logical Operator14/2
  [VINP_BMSWarn6_flg] -> Logical Operator11/1
  VDDM_C3BMS6LCCFS_flg/1 -> [VDDM_C3BMS6LCCFS_flg]
  VINP_MCUWarnF_enum/1 -> [VINP_MCUWarnF_enum]
  VDDM_MCUF1NoComCFS_flg/1 -> [VDDM_MCUF1NoComCFS_flg]
  VDDM_MCUR1NoComCFS_flg/1 -> [VDDM_MCUR1NoComCFS_flg]
  VINP_MCUWarnR_enum/1 -> [VINP_MCUWarnR_enum]
  VPMM_DrivetrainSelect_enum/1 -> [VPMM_DrivetrainSelect_enum]
  VPMM_PowerSta_enum/1 -> [VPMM_PowerSta_enum]
  VPMM_PwrStaSW_enum/1 -> [VPMM_PwrStaSW_enum]
  task_time_s/1 -> [task_time_s]
  VINP_BMSWarn6_flg/1 -> [VINP_BMSWarn6_flg]

== system ddm/DDM/DDM/PMM/Fault level/Fault level 4 subsystem error ==
  note: Diagnostics and Fault Handling
  note: Fail Safe Operation After Failure Decision
  note: Test Pass Criteria
  note: Release Condition During Failure Detection
  note: Release Condition After Failure Decision
  note: Test Detection Criteria
  note: Fail Safe Operation During Failure Detection
  task_time_s : Inport
  VPMM_PowerSta_enum : Inport  Port=2
  VPMM_PwrStaSW_enum : Inport  Port=3
  VDDM_C3BMS6LCCFS_flg : Inport  Port=4
  VINP_BMSWarn7_flg : Inport  Port=5
  VINP_BMSWarn8_flg : Inport  Port=6
  DTC_clear_request : Inport  Port=7
  No_CAN3_BUS_OFF : Inport  Port=8
  Constant10 : Constant  Value=KDDM_Lv4ErrDetSW_flg
  Constant11 : Constant  Value=KDDM_Lv4ErrPassSW_flg
  Constant15 : Constant  Value=KDDM_Lv4ErrCFSSW_flg
  Constant16 : Constant  Value=TRUE
  Constant18 : Constant  Value=KDDM_Lv4ErrPassTO_s
  Constant19 : Constant  Value=ENUM_POWERSTA_OFF
  Constant{2,21,25,27} (4 alike) : Constant  Value=FALSE
  Constant20 : Constant  Value=KDDM_Lv4ErrDFSSW_flg
  Constant22 : Constant  Value=ENUM_PWRSTASW_OFF
  Constant23 : Constant  Value=TRUE
  Constant24 : Constant  Value=TRUE
  Constant26 : Constant  Value=ENUM_PWRSTASW_OFF
  Constant3 : Constant  Value=KDDM_Lv4ErrDetTO_s
  Constant4 : Constant  Value=KDDM_Lv4ErrPassTO_s
  Constant40 : Constant  Value=KDDM_Lv4ErrDTC_cnt
  Constant5 : Constant  Value=KDDM_Lv4ErrDTC_cnt
  DTC_Couter : hcu_lib/Basic_Blocks/DTC_Couter
  DTC_Info : hcu_lib/Basic_Blocks/DTC_Info
  Data Type Conversion1 : DataTypeConversion  OutDataTypeStr=uint8
  Equal : RelationalOperator  Operator=~=  OutDataTypeStr=boolean  RndMeth=Simplest
  Equal2 : RelationalOperator  Operator=~=  OutDataTypeStr=boolean  RndMeth=Simplest
  Equal3 : RelationalOperator  OutDataTypeStr=boolean  RndMeth=Simplest
  Equal4 : RelationalOperator  Operator===  OutDataTypeStr=boolean  RndMeth=Simplest
  Goto24 : Goto  Commented=on  GotoTag=VDDM_EDriveSysErrVCUErr_flg
  Logical Operator{1,4,6,9} (4 alike) : Logic  Operator=NOT  AllPortsSameDT=off  OutDataTypeStr=boolean
  Logical Operator{5,8,10..11,13} (5 alike) : Logic  Operator=OR  AllPortsSameDT=off  OutDataTypeStr=boolean
  Logical Operator12 : Logic  AllPortsSameDT=off  OutDataTypeStr=boolean
  Logical Operator15 : Logic  AllPortsSameDT=off  OutDataTypeStr=boolean
  Logical Operator18 : Logic  AllPortsSameDT=off  OutDataTypeStr=boolean
  Logical Operator19 : Logic  Inputs=3  AllPortsSameDT=off  OutDataTypeStr=boolean
  Logical Operator2 : Logic  Inputs=3  AllPortsSameDT=off  OutDataTypeStr=boolean
  Logical Operator3 : Logic  Operator=OR  Inputs=3  AllPortsSameDT=off  OutDataTypeStr=boolean
  Logical Operator7 : Logic  Inputs=3  AllPortsSameDT=off  OutDataTypeStr=boolean
  Relay : Relay  OnSwitchValue=ONE_INT  OffSwitchValue=ZERO_INT
  SR_Latch1 : Subsystem  mask(SR_Latch){}
      mask help: SR latch function.
  SR_Latch3 : hcu_lib/Basic_Blocks/SR_Latch
  SR_Latch4 : hcu_lib/Basic_Blocks/SR_Latch
  Switch{,2,4..6} (5 alike) : Switch  Criteria=u2 ~= 0
  Test Detection Criteria : hcu_lib/Basic_Blocks/Test Detection Criteria
  Timer1 : hcu_lib/Basic_Blocks/Timer
  VDDM_Lv4ErrDTC_raw32 : Outport
  wires:
  [DTC_clear_request] -> Logical Operator10/2
  DTC_Couter/2 -> Data Type Conversion1/1
  Logical Operator12/1 -> [VDDM_Lv4ErrDFS_flg]  "VDDM_Lv4ErrDFS_flg"
  Constant11/1 -> Logical Operator15/2
  [VDDM_Lv4ErrCFS_flg] -> Logical Operator13/1
  [VDDM_Lv4ErrPass_flg] -> Logical Operator3/1
  Logical Operator18/1 -> [VDDM_Lv4ErrCFS_flg]  "VDDM_Lv4ErrCFS_flg"
  Constant15/1 -> Logical Operator18/2
  [VDDM_Lv4ErrCFSRls_flg] -> Logical Operator10/1
  [VDDM_Lv4ErrDTC_cnt] -> Relay/1
  [DTC_clear_request] -> Logical Operator9/1
  Relay/1 -> SR_Latch3/1
  Logical Operator3/1 -> Logical Operator15/1
  Logical Operator19/1 -> DTC_Couter/1
  Data Type Conversion1/1 -> [VDDM_Lv4ErrDTC_cnt]  "VDDM_Lv4ErrDTC_cnt"
  SR_Latch3/1 -> Logical Operator12/2
  Constant5/1 -> DTC_Couter/3
  [VDDM_Lv4ErrDet_flg] -> Logical Operator19/1
  Logical Operator15/1 -> DTC_Couter/2
  DTC_Couter/1 -> SR_Latch4/1
  [DTC_clear_request] -> Logical Operator3/3
  Constant10/1 -> Logical Operator19/2
  SR_Latch4/1 -> Logical Operator18/1
  Logical Operator9/1 -> Logical Operator19/3
  [DTC_clear_request] -> Logical Operator13/2
  Logical Operator10/1 -> SR_Latch4/2
  Logical Operator13/1 -> SR_Latch3/2
  Constant20/1 -> Logical Operator12/1
  [VDDM_Lv4ErrCFSRls_flg] -> Logical Operator3/2
  [VDDM_xxx_flg] -> SR_Latch1/2(reset)
  Constant2/1 -> Switch6/1
  Switch5/1 -> Switch6/3, [VDDM_xxx_flg]
  Switch6/1 -> Test Detection Criteria/1
  [DTC_clear_request] -> Switch6/2
  [DTC_clear_request] -> DTC_Info/4
  Constant3/1 -> Test Detection Criteria/4
  [VDDM_Lv4ErrDet_flg] -> DTC_Info/1
  [VDDM_Lv4ErrCFS_flg] -> DTC_Info/3
  [VDDM_Lv4ErrPass_flg] -> DTC_Info/2
  DTC_Info/1 -> VDDM_Lv4ErrDTC_raw32/1  "VDDM_Lv4ErrDTC_raw32"
  [task_time_s] -> Timer1/3
  No_CAN3_BUS_OFF/1 -> [No_CAN3_BUS_OFF]
  DTC_clear_request/1 -> [DTC_clear_request]
  [VPMM_PwrStaSW_enum] -> Equal/1
  [VPMM_PowerSta_enum] -> Equal4/1
  [VINP_BMSWarn7_flg] -> Logical Operator5/1
  [No_CAN3_BUS_OFF] -> Logical Operator7/1
  [VDDM_C3BMS6LCCFS_flg] -> Logical Operator4/1
  [VPMM_PwrStaSW_enum] -> Equal2/1
  Logical Operator4/1 -> Logical Operator7/3
  Logical Operator7/1 -> Switch2/2
  Constant22/1 -> Equal2/2
  Constant23/1 -> Switch2/3
  Equal2/1 -> Logical Operator7/2
  Logical Operator5/1 -> Switch2/1
  [VINP_BMSWarn8_flg] -> Logical Operator5/2
  [VINP_BMSWarn8_flg] -> Logical Operator11/2
  Constant4/1 -> Timer1/4
  Constant19/1 -> Equal4/2
  Constant25/1 -> Switch4/3
  Logical Operator11/1 -> Switch5/1
  Test Detection Criteria/1 -> [VDDM_Lv4ErrDet_flg]  "VDDM_Lv4ErrDet_flg"
  Constant21/1 -> Switch/3
  Equal/1 -> Logical Operator2/2
  Constant27/1 -> Switch5/3
  Switch4/1 -> [VDDM_Lv4ErrCFSRls_flg]  "VDDM_Lv4ErrCFSRls_flg"
  Constant16/1 -> Switch/1
  Logical Operator8/1 -> Switch4/2
  Switch2/1 -> Timer1/2, Logical Operator6/1
  Logical Operator2/1 -> Switch5/2
  Constant24/1 -> Switch4/1
  Logical Operator1/1 -> Logical Operator2/3
  Constant18/1 -> Equal3/2
  Constant26/1 -> Equal/2
  Timer1/1 -> Equal3/1
  [DTC_clear_request] -> Logical Operator8/2
  Equal4/1 -> Logical Operator8/1
  Constant40/1 -> Test Detection Criteria/3
  Equal3/1 -> SR_Latch1/1(set)
  Switch/1 -> Goto24/1
  [VDDM_C3BMS6LCCFS_flg] -> Logical Operator1/1
  [VDDM_Lv4ErrCFS_flg] -> Switch/2
  [task_time_s] -> Test Detection Criteria/2
  Logical Operator6/1 -> Timer1/1
  [No_CAN3_BUS_OFF] -> Logical Operator2/1
  [VINP_BMSWarn7_flg] -> Logical Operator11/1
  SR_Latch1/1(latched) -> [VDDM_Lv4ErrPass_flg]  "VDDM_Lv4ErrPass_flg"
  VDDM_C3BMS6LCCFS_flg/1 -> [VDDM_C3BMS6LCCFS_flg]
  VINP_BMSWarn7_flg/1 -> [VINP_BMSWarn7_flg]
  task_time_s/1 -> [task_time_s]
  VPMM_PwrStaSW_enum/1 -> [VPMM_PwrStaSW_enum]
  VPMM_PowerSta_enum/1 -> [VPMM_PowerSta_enum]
  VINP_BMSWarn8_flg/1 -> [VINP_BMSWarn8_flg]

== system ddm/DDM/DDM/PMM/Key authentication failed/SR_Latch1 ==
  set : Inport
  reset : Inport  Port=2
  Logical Operator : Logic  AllPortsSameDT=off  OutDataTypeStr=boolean
  Logical Operator1 : Logic  Operator=NOT  AllPortsSameDT=off  OutDataTypeStr=boolean
  Switch1 : Switch  Criteria=u2 ~= 0  Threshold=0.5
      settings: AttributesFormatString=<Criteria=%<Criteria>>
  Switch2 : Switch  Criteria=u2 ~= 0  Threshold=0.5
      settings: AttributesFormatString=<Criteria=%<Criteria>>
  Unit Delay : UnitDelay  SampleTime=-1  HasFrameUpgradeWarning=on
  latched : Outport
  wires:
  Logical Operator1/1 -> Switch2/1, Logical Operator/2
  Logical Operator/1 -> Switch1/2
  Switch2/1 -> Switch1/3
  Unit Delay/1 -> Switch2/3
  reset/1 -> Logical Operator1/1, Switch2/2
  set/1 -> Logical Operator/1, Switch1/1
  Switch1/1 -> latched/1, Unit Delay/1

== system ddm/DDM/DDM/PMM/LV/Initial LV battery voltage too low ==
  note: Diagnostics and Fault Handling
  note: Release Condition After Decision
  note: Release Condition During Detection
  note: Fail Safe During Detection
  note: Fail Safe After Decision
  note: Test Pass Criteria
  note: Test Detection Criteria
  task_time_s : Inport
  VPMM_PowerSta_enum : Inport  Port=2
  VPMM_PwrStaSW_enum : Inport  Port=3
  VINP_LVBattDet12V_V : Inport  Port=4
  VINP_CANMsgValidBMS2_flg : Inport  Port=5
  DTC_clear_request : Inport  Port=6
  Constant1 : Constant  Value=TRUE
  Constant10 : Constant  Value=ENUM_POWERSTA_OFF
  Constant11 : Constant  Value=KDDM_IniLVLoPassSW_flg
  Constant15 : Constant  Value=KDDM_IniLVLoCFSSW_flg
  Constant16 : Constant  Value=TRUE
  Constant18 : Constant  Value=KDDM_IniLVLoPassTO_s
  Constant19 : Constant  Value=KDDM_IniLVLoPassTO_s
  Constant2 : Constant  Value=ENUM_PWRSTASW_STANDBY
  Constant20 : Constant  Value=KDDM_IniLVLoDFSSW_flg
  Constant{4,8,21,25} (4 alike) : Constant  Value=FALSE
  Constant24 : Constant  Value=TRUE
  Constant3 : Constant  Value=ENUM_PWRSTASW_OFF
  Constant40 : Constant  Value=KDDM_IniLVLoDTC_cnt
  Constant41 : Constant  Value=KDDM_IniLVLoDetTO_s
  Constant46 : Constant  Value=KDDM_IniLVLoDetSW_flg
  Constant48 : Constant  Value=KDDM_IniLVLoDTC_cnt
  Constant5 : Constant  Value=ENUM_PWRSTASW_STANDBY
  Constant6 : Constant  Value=KDDM_IniLVLoThd_mv
  Constant7 : Constant  Value=ENUM_PWRSTASW_OFF
  Constant9 : Constant  Value=KDDM_IniLVLoThd_mv
  DTC_Couter : hcu_lib/Basic_Blocks/DTC_Couter
  DTC_Info : hcu_lib/Basic_Blocks/DTC_Info
  Data Type Conversion1 : DataTypeConversion  OutDataTypeStr=uint8
  Equal{,1..2,4,6} (5 alike) : RelationalOperator  Operator===  OutDataTypeStr=boolean  RndMeth=Simplest
  Equal3 : RelationalOperator  OutDataTypeStr=boolean  RndMeth=Simplest
  Equal5 : RelationalOperator  Operator=<=  OutDataTypeStr=boolean  RndMeth=Simplest
  Equal7 : RelationalOperator  Operator=<=  OutDataTypeStr=boolean  RndMeth=Simplest
  Gain1 : Gain  Gain=1000
  Gain2 : Gain  Gain=1000
  Goto6 : Goto  Commented=on  GotoTag=VDDM_EDriveSysErrVCUErr_flg
  Logical Operator{1..2,12,15,18} (5 alike) : Logic  AllPortsSameDT=off  OutDataTypeStr=boolean
  Logical Operator19 : Logic  Inputs=3  AllPortsSameDT=off  OutDataTypeStr=boolean
  Logical Operator3 : Logic  Operator=OR  Inputs=3  AllPortsSameDT=off  OutDataTypeStr=boolean
  Logical Operator4 : Logic  Operator=NOT  AllPortsSameDT=off  OutDataTypeStr=boolean
  Logical Operator5 : Logic  Operator=OR  AllPortsSameDT=off  OutDataTypeStr=boolean
  Logical Operator6 : Logic  Operator=NOT  AllPortsSameDT=off  OutDataTypeStr=boolean
  Logical Operator7 : Logic  Operator=OR  AllPortsSameDT=off  OutDataTypeStr=boolean
  Logical Operator8 : Logic  Operator=OR  AllPortsSameDT=off  OutDataTypeStr=boolean
  OR : Logic  Operator=OR  AllPortsSameDT=off  OutDataTypeStr=boolean
  OR1 : Logic  Operator=OR  AllPortsSameDT=off  OutDataTypeStr=boolean
  Relay : Relay  OnSwitchValue=ONE_INT  OffSwitchValue=ZERO_INT
  SR_Latch1 : Subsystem  mask(SR_Latch){}
      mask help: SR latch function.
  SR_Latch3 : hcu_lib/Basic_Blocks/SR_Latch
  SR_Latch4 : hcu_lib/Basic_Blocks/SR_Latch
  Switch{,2..4,6} (5 alike) : Switch  Criteria=u2 ~= 0
  Test Detection Criteria : hcu_lib/Basic_Blocks/Test Detection Criteria
  Timer1 : hcu_lib/Basic_Blocks/Timer
  VDDM_IniLVLoDTC_raw32 : Outport
  wires:
  DTC_Couter/1 -> SR_Latch4/1
  [VDDM_IniLVLoDet_flg] -> Logical Operator19/1
  [VDDM_IniLVLoPass_flg] -> Logical Operator3/1
  Constant46/1 -> Logical Operator19/2
  [DTC_clear_request] -> Logical Operator5/2
  SR_Latch4/1 -> Logical Operator18/1
  DTC_Couter/2 -> Data Type Conversion1/1
  Logical Operator19/1 -> DTC_Couter/1
  Logical Operator5/1 -> SR_Latch4/2
  Relay/1 -> SR_Latch3/1
  [VDDM_IniLVLoDTC_cnt] -> Relay/1
  [DTC_clear_request] -> Logical Operator3/3
  [VDDM_IniLVLoCFS_flg] -> Logical Operator7/1
  [DTC_clear_request] -> Logical Operator7/2
  [VDDM_IniLVLoCFSRls_flg] -> Logical Operator5/1
  Constant15/1 -> Logical Operator18/2
  Constant20/1 -> Logical Operator12/1
  Logical Operator3/1 -> Logical Operator15/1
  [VDDM_IniLVLoCFSRls_flg] -> Logical Operator3/2
  Constant11/1 -> Logical Operator15/2
  Logical Operator12/1 -> [VDDM_IniLVLoDFS_flg]  "VDDM_IniLVLoDFS_flg"
  Constant48/1 -> DTC_Couter/3
  Logical Operator7/1 -> SR_Latch3/2
  Logical Operator18/1 -> [VDDM_IniLVLoCFS_flg]  "VDDM_IniLVLoCFS_flg"
  [DTC_clear_request] -> Logical Operator4/1
  Logical Operator4/1 -> Logical Operator19/3
  Data Type Conversion1/1 -> [VDDM_IniLVLoDTC_cnt]  "VDDM_IniLVLoDTC_cnt"
  Logical Operator15/1 -> DTC_Couter/2
  SR_Latch3/1 -> Logical Operator12/2
  [VDDM_xxx_flg] -> SR_Latch1/2(reset)
  Constant8/1 -> Switch6/1
  Switch3/1 -> Switch6/3, [VDDM_xxx_flg]
  Switch6/1 -> Test Detection Criteria/1
  [DTC_clear_request] -> Switch6/2
  [DTC_clear_request] -> DTC_Info/4
  Constant41/1 -> Test Detection Criteria/4
  [VDDM_IniLVLoDet_flg] -> DTC_Info/1
  [VDDM_IniLVLoCFS_flg] -> DTC_Info/3
  [VDDM_IniLVLoPass_flg] -> DTC_Info/2
  DTC_Info/1 -> VDDM_IniLVLoDTC_raw32/1  "VDDM_IniLVLoDTC_raw32"
  [VPMM_PowerSta_enum] -> Equal4/1
  [task_time_s] -> Timer1/3
  Constant5/1 -> Equal6/1
  Equal2/1 -> OR1/2
  OR1/1 -> Logical Operator1/1
  Constant9/1 -> Equal7/2
  [VINP_LVBattDet12V_V] -> Gain2/1
  Gain2/1 -> Equal7/1
  Constant7/1 -> Equal2/2
  Logical Operator1/1 -> Switch4/2
  Equal6/1 -> OR1/1
  [VPMM_PwrStaSW_enum] -> Equal2/1, Equal6/2
  [VINP_CANMsgValidBMS2_flg] -> Logical Operator1/2
  Equal7/1 -> Switch4/1
  Gain1/1 -> Equal5/1
  Constant6/1 -> Equal5/2
  Equal5/1 -> Switch3/1
  [VINP_LVBattDet12V_V] -> Gain1/1
  Constant2/1 -> Equal1/1
  Equal1/1 -> OR/1
  OR/1 -> Logical Operator2/1
  Equal/1 -> OR/2
  [VINP_CANMsgValidBMS2_flg] -> Logical Operator2/2
  VINP_CANMsgValidBMS2_flg/1 -> [VINP_CANMsgValidBMS2_flg]
  DTC_clear_request/1 -> [DTC_clear_request]
  Equal4/1 -> Logical Operator8/1
  Constant10/1 -> Equal4/2
  Constant24/1 -> Switch2/1
  [DTC_clear_request] -> Logical Operator8/2
  Switch2/1 -> [VDDM_IniLVLoCFSRls_flg]  "VDDM_IniLVLoCFSRls_flg"
  Constant25/1 -> Switch2/3
  Logical Operator8/1 -> Switch2/2
  Constant21/1 -> Switch/3
  Constant1/1 -> Switch/1
  Switch/1 -> Goto6/1
  [VDDM_IniLVLoCFS_flg] -> Switch/2
  Constant16/1 -> Switch4/3
  Constant18/1 -> Timer1/4
  Timer1/1 -> Equal3/1
  Switch4/1 -> Timer1/2, Logical Operator6/1
  Constant19/1 -> Equal3/2
  Logical Operator6/1 -> Timer1/1
  Equal3/1 -> SR_Latch1/1(set)
  SR_Latch1/1(latched) -> [VDDM_IniLVLoPass_flg]  "VDDM_IniLVLoPass_flg"
  [VPMM_PwrStaSW_enum] -> Equal/1, Equal1/2
  Constant4/1 -> Switch3/3
  Constant3/1 -> Equal/2
  Constant40/1 -> Test Detection Criteria/3
  Test Detection Criteria/1 -> [VDDM_IniLVLoDet_flg]  "VDDM_IniLVLoDet_flg"
  [task_time_s] -> Test Detection Criteria/2
  Logical Operator2/1 -> Switch3/2
  VPMM_PowerSta_enum/1 -> [VPMM_PowerSta_enum]
  VPMM_PwrStaSW_enum/1 -> [VPMM_PwrStaSW_enum]
  VINP_LVBattDet12V_V/1 -> [VINP_LVBattDet12V_V]
  task_time_s/1 -> [task_time_s]
